simulink model "Three_ph_IM_speed_control"  (R2024b)
settings: Solver=VariableStepAuto  StartTime=0.0  StopTime=1  RelTol=1e-3
libraries: spsSeriesRLCBranchLib x9, spsThyristorLib x6, spsVoltageMeasurementLib x6, spsGroundLib x4, spsACVoltageSourceLib x3, spsRMSLib x2, spsAsynchronousMachineSIUnitsLib x1, sps_lib x1
settings Model: Creator=hp  LastModifiedBy=hp

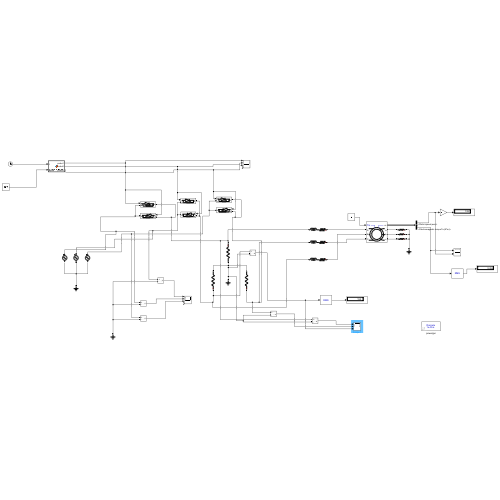
[thumbnail: Simulink's stored preview of the top-level diagram]
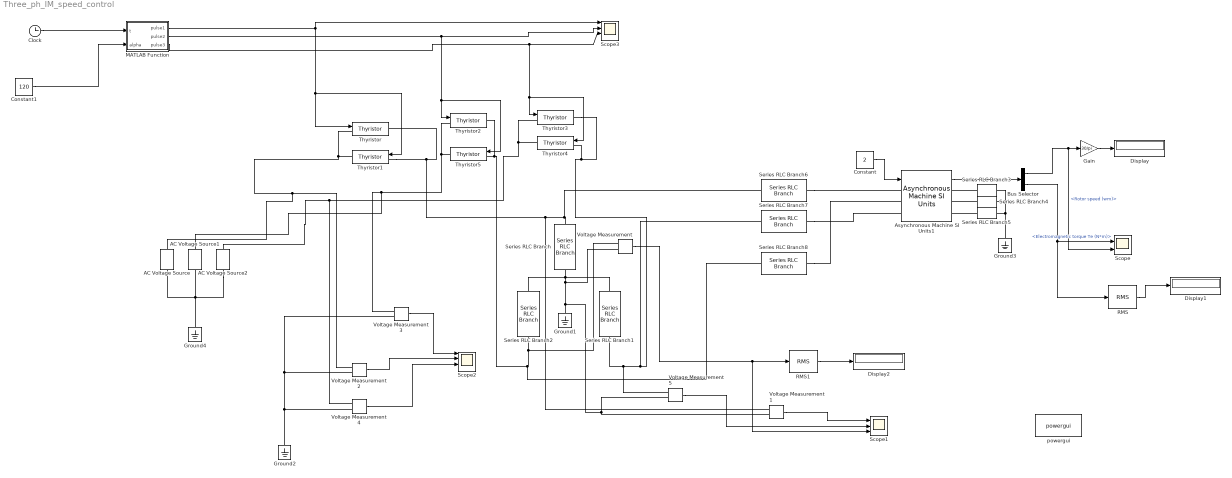
== system Three_ph_IM_speed_control ==
  AC Voltage Source : spsACVoltageSourceLib/AC Voltage Source  Amplitude=340  Phase=0  Frequency=50  SampleTime=0  Measurements=None  BusType=PV  Pref=6000  Qref=0  Qmin=-inf  Qmax=+inf
  AC Voltage Source1 : spsACVoltageSourceLib/AC Voltage Source  Amplitude=340  Phase=-120  Frequency=50  SampleTime=0  Measurements=None  BusType=PV  Pref=6000  Qref=0  Qmin=-inf  Qmax=+inf
  AC Voltage Source2 : spsACVoltageSourceLib/AC Voltage Source  Amplitude=340  Phase=120  Frequency=50  SampleTime=0  Measurements=None  BusType=PV  Pref=6000  Qref=0  Qmin=-inf  Qmax=+inf
  Asynchronous Machine SI Units1 : spsAsynchronousMachineSIUnitsLib/Asynchronous Machine SI Units  RotorType=Wound  PresetModel=No  MechanicalLoad=Torque Tm  ShowDetailedParameters=on  ReferenceFrame=Rotor  Units=SI  MeasurementBus=off  NominalParameters=[2000 400 50]  VoltageRatio=1  Stator=[1.405 0.005839]  Rotor=[1.395 0.005839]  Cage1=[0.4155 0.002066]  Cage2=[0.4168 0.0003495]  Lm=0.1722  Mechanical=[0.0131 0.002985 2]  PolePairs=2  InitialConditions=[0 0 0 0 0 0 0 0]  SimulateSaturation=off  Saturation=[14.03593122, 27.81365428, 53.79336849, 72.68890987, 97.98006896, 148.6815601, 215.7428561, 302.9841135, 428.7778367 ; 230, 322, 414, 460, 506, 552, 598, 644, 690]  LoadFlowParameters=1492000  TsPowergui=0  TsBlock=-1  IterativeModel=Trapezoidal non iterative  IterativeDiscreteModel=Trapezoidal robust  Pmec=1500
  Bus Selector : BusSelector  OutputSignals=Mechanical.Rotor speed (wm),Mechanical.Electromagnetic torque Te (N*m)
  Clock : Clock
  Constant : Constant  Value=2
  Constant1 : Constant  Value=120
  Display : Display
  Display1 : Display
  Display2 : Display
  Gain : Gain  Gain=30/pi
  Ground{1..4} (4 alike) : spsGroundLib/Ground  LConnTagsString=a
  MATLAB Function : MATLAB Function  TreatAsAtomicUnit=on
  RMS : spsRMSLib/RMS  TrueRMS=on  Freq=60  RMSInit=120  Ts=0
  RMS1 : spsRMSLib/RMS  TrueRMS=on  Freq=60  RMSInit=120  Ts=0
  Scope : Scope  NumInputPorts=2
  Scope1 : Scope  NumInputPorts=3
  Scope2 : Scope  NumInputPorts=4
  Scope3 : Scope  NumInputPorts=4
  Series RLC Branch : spsSeriesRLCBranchLib/Series RLC Branch  LConnTagsString=__new0  RConnTagsString=__new0  BranchType=R  Resistance=100  Inductance=1e-3  SetiL0=off  InitialCurrent=0  Capacitance=1e-6  Setx0=off  InitialVoltage=0  Measurements=None
  Series RLC Branch1 : spsSeriesRLCBranchLib/Series RLC Branch  LConnTagsString=__new0  RConnTagsString=__new0  BranchType=R  Resistance=100  Inductance=1e-3  SetiL0=off  InitialCurrent=0  Capacitance=1e-6  Setx0=off  InitialVoltage=0  Measurements=None
  Series RLC Branch2 : spsSeriesRLCBranchLib/Series RLC Branch  LConnTagsString=__new0  RConnTagsString=__new0  BranchType=R  Resistance=100  Inductance=1e-3  SetiL0=off  InitialCurrent=0  Capacitance=1e-6  Setx0=off  InitialVoltage=0  Measurements=None
  Series RLC Branch3 : spsSeriesRLCBranchLib/Series RLC Branch  LConnTagsString=__new0  RConnTagsString=__new0  BranchType=R  Resistance=2  Inductance=1e-3  SetiL0=off  InitialCurrent=0  Capacitance=1e-6  Setx0=off  InitialVoltage=0  Measurements=None
  Series RLC Branch4 : spsSeriesRLCBranchLib/Series RLC Branch  LConnTagsString=__new0  RConnTagsString=__new0  BranchType=R  Resistance=2  Inductance=1e-3  SetiL0=off  InitialCurrent=0  Capacitance=1e-6  Setx0=off  InitialVoltage=0  Measurements=None
  Series RLC Branch5 : spsSeriesRLCBranchLib/Series RLC Branch  LConnTagsString=__new0  RConnTagsString=__new0  BranchType=R  Resistance=2  Inductance=1e-3  SetiL0=off  InitialCurrent=0  Capacitance=1e-6  Setx0=off  InitialVoltage=0  Measurements=None
  Series RLC Branch6 : spsSeriesRLCBranchLib/Series RLC Branch  LConnTagsString=__new0  RConnTagsString=__new0  BranchType=RL  Resistance=5  Inductance=1e-3  SetiL0=off  InitialCurrent=0  Capacitance=1e-6  Setx0=off  InitialVoltage=0  Measurements=None
  Series RLC Branch7 : spsSeriesRLCBranchLib/Series RLC Branch  LConnTagsString=__new0  RConnTagsString=__new0  BranchType=RL  Resistance=5  Inductance=1e-3  SetiL0=off  InitialCurrent=0  Capacitance=1e-6  Setx0=off  InitialVoltage=0  Measurements=None
  Series RLC Branch8 : spsSeriesRLCBranchLib/Series RLC Branch  LConnTagsString=__new0  RConnTagsString=__new0  BranchType=RL  Resistance=5  Inductance=1e-3  SetiL0=off  InitialCurrent=0  Capacitance=1e-6  Setx0=off  InitialVoltage=0  Measurements=None
  Thyristor{,1..5} (6 alike) : spsThyristorLib/Thyristor  Ron=0.001  Lon=0  Vf=0.8  IC=0  Rs=1000  Cs=1*1e-9  Measurements=off
  Voltage Measurement{,1..5} (6 alike) : spsVoltageMeasurementLib/Voltage Measurement  PhasorSimulation=off  OutputType=Complex  PSBequivalent=0
  powergui : sps_lib/powergui  Priority=1  SimulationMode=Discrete  SampleTime=1e-5  frequency=60  Iterations=50  frequencyindice=50  Pbase=100e6  ErrMax=1e-4  UnitsV=kV  UnitsW=MW  buscounter=0  FunctionMessages=off  echomessages=off  EnableUseOfTLC=off  CurrentSourceSwitches=off  DisableSnubberDevices=off  DisableRonSwitches=off  DisableVfSwitches=off  DisplayEquations=off  AutomaticDiscreteSolvers=off  SolverType=Tustin/Backward Euler (TBE)  Interpol=off  ExternalGateDelay=off  methode=off  Ts=100  x0status=blocks  SPID=on  SwTol=0  HookPort=off  NonlinearTolerance=1e-4  nMaxIteration=100  ContinueOnMaxIteration=off  RestoreLinks=warning  ResistiveCurrentMeasurement=off  Frange=[0:2:500]  Ylog=off  Xlog=on  ShowGrid=off  save=off  variable=ZData  structure=0  ZoomFFT=off  StartTime=0.0  cycles=1  DisplayStyle=1  fundamental=60  FreqAxis=off  MaxFrequency=1000  frequencyindicesteady=1  RmsSteady=1  display=off
  wires:
  Voltage Measurement/1 -> Scope1/3, RMS1/1
  RMS1/1 -> Display2/1
  Constant1/1 -> MATLAB Function/2(alpha)
  Voltage Measurement1/1 -> Scope1/1
  Voltage Measurement5/1 -> Scope1/2
  Voltage Measurement4/1 -> Scope2/3
  Voltage Measurement2/1 -> Scope2/2
  Voltage Measurement3/1 -> Scope2/1
  Clock/1 -> MATLAB Function/1(t)
  MATLAB Function/1(pulse1) -> Scope3/1, Thyristor1/1, Thyristor/1
  MATLAB Function/2(pulse2) -> Scope3/2, Thyristor5/1, Thyristor2/1
  MATLAB Function/3(pulse3) -> Thyristor4/1, Thyristor3/1, Scope3/3
  Gain/1 -> Display/1
  Constant/1 -> Asynchronous Machine SI Units1/1
  RMS/1 -> Display1/1
  Asynchronous Machine SI Units1/1 -> Bus Selector/1
  Bus Selector/2 -> RMS/1, Scope/1  "<Electromagnetic torque Te (N*m)>"
  Bus Selector/1 -> Scope/2, Gain/1  "<Rotor speed (wm)>"
  connections:
  Thyristor1/LConn1 -- Thyristor/RConn1 -- Voltage Measurement1/LConn1 -- Series RLC Branch6/RConn1 -- Series RLC Branch/LConn1
  Thyristor3/RConn1 -- Series RLC Branch7/RConn1 -- Series RLC Branch1/LConn1 -- Voltage Measurement5/LConn1 -- Thyristor4/LConn1
  Thyristor2/LConn1 -- Voltage Measurement3/LConn1 -- AC Voltage Source1/RConn1 -- Thyristor5/RConn1
  Thyristor3/LConn1 -- AC Voltage Source2/RConn1 -- Voltage Measurement4/LConn1 -- Thyristor4/RConn1
  Series RLC Branch2/RConn1 -- Voltage Measurement5/LConn2 -- Voltage Measurement1/LConn2 -- Ground1/LConn1 -- Voltage Measurement/LConn2 -- Series RLC Branch1/RConn1 -- Series RLC Branch/RConn1
  Voltage Measurement2/LConn2 -- Ground2/LConn1 -- Voltage Measurement4/LConn2 -- Voltage Measurement3/LConn2
  Thyristor/LConn1 -- Voltage Measurement2/LConn1 -- AC Voltage Source/RConn1 -- Thyristor1/RConn1
  AC Voltage Source2/LConn1 -- Ground4/LConn1 -- AC Voltage Source/LConn1 -- AC Voltage Source1/LConn1
  Thyristor2/RConn1 -- Series RLC Branch8/RConn1 -- Voltage Measurement/LConn1 -- Series RLC Branch2/LConn1 -- Thyristor5/LConn1
  Series RLC Branch7/LConn1 -- Asynchronous Machine SI Units1/LConn3
  Series RLC Branch6/LConn1 -- Asynchronous Machine SI Units1/LConn1
  Series RLC Branch8/LConn1 -- Asynchronous Machine SI Units1/LConn2
  Series RLC Branch3/RConn1 -- Asynchronous Machine SI Units1/RConn1
  Series RLC Branch4/RConn1 -- Asynchronous Machine SI Units1/RConn2
  Series RLC Branch5/RConn1 -- Asynchronous Machine SI Units1/RConn3
  Series RLC Branch3/LConn1 -- Ground3/LConn1 -- Series RLC Branch5/LConn1 -- Series RLC Branch4/LConn1

== matlab function Three_ph_IM_speed_control/MATLAB Function ==
  data: t input; pulse1 output; alpha input; pulse2 output; pulse3 output
function [pulse1, pulse2, pulse3] = generatePulses(t, alpha)
% Inputs:
%   t     - simulation time (from Simulink clock)
%   alpha - firing angle in degrees (0 to 180 typically)
% Outputs:
%   pulse1, pulse2, pulse3 - three output pulses (0 or 1)

% Constants
f = 100;                  % Frequency in Hz
T = 1 / f;                % Period in seconds
alpha_time = (alpha / 360) *0.02;  % Convert firing angle to time delay

% Pulse width (adjustable)
pulse_width = 0.0020;     % 500 µs wide pulse

% Time in current cycle
t_mod = mod(t, T);

% Pulse start times (120° = T/3 apart)
start1 = alpha_time;
start2 = mod(alpha_time + 2*T/3, T);   % +120°
start3 = mod(alpha_time + T/3, T); % +240°

% Generate pulses
pulse1 = double(t_mod >= start1-pulse_width/2 && t_mod <= start1 + pulse_width/2);
pulse2 = double(t_mod >= start2-pulse_width/2 && t_mod <= start2 + pulse_width/2);
pulse3 = double(t_mod >= start3-pulse_width/2 && t_mod <= start3 + pulse_width/2);
